simulink model "PHIL_GFMI"  (R2016a)
settings: Solver=FixedStepDiscrete  StartTime=0.0  StopTime=150  FixedStep=0.001  RelTol=1e-3
libraries: powerlib_meascontrol x2
settings Model: Creator=CoSES_HPC2  LastModifiedBy=CoSES_HPC2
settings DebuggingCC: RootOutportRequireBusObject=error  StrictBusMsg=ErrorOnBusTreatedAsVector
settings HardwareCC: ProdBitPerPointer=32  ProdLargestAtomicFloat=None  ProdWordSize=32  ProdHWDeviceType=Intel->x86/Pentium
settings RTWCC: SystemTargetFile=NIVeriStand.tlc  TemplateMakefile=NIVeriStand_vc.tmf  Description=NI Phar Lap Real-Time & Windows Targets
settings STFCustomTargetCC: MatFileLogging=on  SystemTargetFile=NIVeriStand.tlc
settings GRTTargetCC: ParMdlRefBuildCompliant=off  CompOptLevelCompliant=off  ConcurrentExecutionCompliant=off  GeneratePreprocessorConditionals=Use local settings  CombineOutputUpdateFcns=off  CPPClassGenCompliant=off  GRTInterface=on  UseToolchainInfoCompliant=off

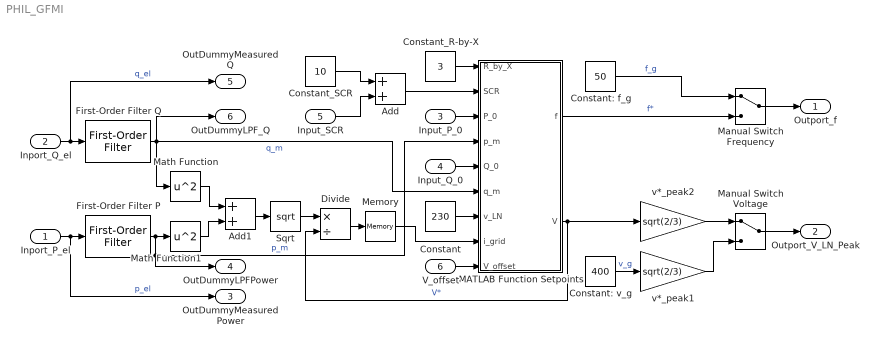
== system PHIL_GFMI ==
  Inport_P_el : Inport
  Inport_Q_el : Inport  Port=2
  Input_P_0 : Inport  Port=3
  Input_Q_0 : Inport  Port=4
  Input_SCR : Inport  Port=5
  V_offset : Inport  Port=6
  Add : Sum
  Add1 : Sum
  Constant : Constant  Value=230
  Constant: f_g : Constant  Value=50
  Constant: v_g : Constant  Value=400
  Constant_R-by-X : Constant  Value=3
  Constant_SCR : Constant  Value=10
  Divide : Product  Inputs=*/
  First-Order Filter P : powerlib_meascontrol/Filters/First-Order Filter  FilterType=Lowpass  Tc=1  Ts=1e-3  Initialize=on  Vac_Init=[0,0,0]  Vdc_Init=0  PlotResponse=off  FreqRange="[0,  200,  1]"
  First-Order Filter Q : powerlib_meascontrol/Filters/First-Order Filter  FilterType=Lowpass  Tc=1  Ts=1e-3  Initialize=on  Vac_Init=[0,0,0]  Vdc_Init=0  PlotResponse=off  FreqRange="[0,  200,  1]"
  MATLAB Function Setpoints : MATLAB Function  TreatAsAtomicUnit=on
  Manual Switch Frequency : ManualSwitch
  Manual Switch Voltage : ManualSwitch
  Math Function : Math  Operator=square  SaturateOnIntegerOverflow=on
  Math Function1 : Math  Operator=square  SaturateOnIntegerOverflow=on
  Memory : Memory
  Sqrt : Sqrt  SaturateOnIntegerOverflow=on
  v*_peak1 : Gain  Gain=sqrt(2/3)
  v*_peak2 : Gain  Gain=sqrt(2/3)
  Outport_f : Outport
  Outport_V_LN_Peak : Outport  Port=2
  OutDummyMeasuredPower : Outport  Port=3
  OutDummyLPFPower : Outport  Port=4
  OutDummyMeasuredQ : Outport  Port=5
  OutDummyLPF_Q : Outport  Port=6
  wires:
  Constant: f_g/1 -> Manual Switch Frequency/1  "f_g"
  First-Order Filter P/1 -> OutDummyLPFPower/1, MATLAB Function Setpoints/4(p_m), Math Function1/1  "p_m"
  Inport_Q_el/1 -> OutDummyMeasuredQ/1, First-Order Filter Q/1  "q_el"
  v*_peak1/1 -> Manual Switch Voltage/2
  Inport_P_el/1 -> OutDummyMeasuredPower/1, First-Order Filter P/1  "p_el"
  Manual Switch Voltage/1 -> Outport_V_LN_Peak/1
  Manual Switch Frequency/1 -> Outport_f/1
  Constant: v_g/1 -> v*_peak1/1  "v_g"
  MATLAB Function Setpoints/2(V) -> v*_peak2/1, Divide/2  "V*"
  MATLAB Function Setpoints/1(f) -> Manual Switch Frequency/2  "f*"
  Input_Q_0/1 -> MATLAB Function Setpoints/5(Q_0)
  First-Order Filter Q/1 -> OutDummyLPF_Q/1, MATLAB Function Setpoints/6(q_m), Math Function/1  "q_m"
  Memory/1 -> MATLAB Function Setpoints/8(i_grid)
  Constant/1 -> MATLAB Function Setpoints/7(v_LN)
  Add/1 -> MATLAB Function Setpoints/2(SCR)
  Constant_SCR/1 -> Add/1
  Input_SCR/1 -> Add/2
  Constant_R-by-X/1 -> MATLAB Function Setpoints/1(R_by_X)
  v*_peak2/1 -> Manual Switch Voltage/1
  V_offset/1 -> MATLAB Function Setpoints/9(V_offset)
  Input_P_0/1 -> MATLAB Function Setpoints/3(P_0)
  Math Function/1 -> Add1/1
  Math Function1/1 -> Add1/2
  Add1/1 -> Sqrt/1
  Sqrt/1 -> Divide/1
  Divide/1 -> Memory/1

== matlab function PHIL_GFMI/MATLAB Function Setpoints ==
  data: f output; R_by_X input; V output; SCR input; P_0 input; p_m input; Q_0 input; q_m input; v_LN input; i_grid input; V_offset input
function [f,V] = fcn(R_by_X, SCR, P_0, p_m, Q_0, q_m, v_LN, i_grid, V_offset)

% Frequency setpoint
f_0 = 50; % Hz
P_b = 10e3; % W
m_p = f_0 * 0.05 / P_b;  % 2.5e-4; 

f = f_0 + m_p * (P_0 - p_m);

% Voltage setpoint
V_0 = 400; % V
S_b = 20e3; % VA
k_q = V_0 * 0.1 / S_b; % 400V * 10% / S_b

deltaV_droop = k_q * ( (R_by_X / sqrt(R_by_X^2 + 1)) * (P_0 - p_m) + (1 / sqrt(R_by_X^2 + 1)) * (Q_0 - q_m) );

Z = v_LN^2 / (S_b * SCR);

deltaV_distance = Z * i_grid;

V = V_0 + deltaV_droop + deltaV_distance + V_offset;
